simulink model "robot_model_stateflow"  (R2024b)
settings: Solver=FixedStepDiscrete  StartTime=0.0  StopTime=10.0  FixedStep=0.1  RelTol=1e-3  EnableMultiTasking=on
settings Model: Creator=ahmed  LastModifiedBy=ahmed
settings SolverCC: AlgebraicLoopSolver=TrustRegion  AutoInsertRateTranBlk=on
settings DataIOCC: LimitDataPoints=on
settings OptimizationCC: LifeSpan=inf
settings DebuggingCC: UnconnectedInputMsg=warning  UnconnectedOutputMsg=warning  UnconnectedLineMsg=warning  AllowSymbolicDim=off  SFUnexpectedBacktrackingDiag=warning  SFNoUnconditionalDefaultTransitionDiag=warning  SFExecutionAtInitializationDiag=none  ArithmeticOperatorsInVariantConditions=warning
settings ModelReferenceCC: EnableRefExpFcnMdlSchedulingChecks=on
settings SFSimCC: SimUseLocalCustomCode=off  CustomCodeUndefinedFunction=UseInterfaceOnly
settings RTWCC: RTWUseLocalCustomCode=off  GPUComputeCapability=3.5  DLArmComputeVersion=19.05
settings CodeAppCC: StateflowObjectComments=on
settings GRTTargetCC: TargetLangStandard=C89/C90 (ANSI)
settings ConfigComp: CovMetricSettings=dw  CovSaveCumulativeToWorkspaceVar=on  CovSaveSingleToWorkspaceVar=on  CovExternalEMLEnable=off

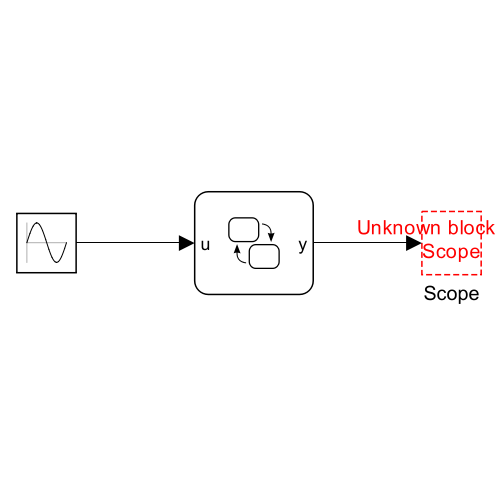
[thumbnail: Simulink's stored preview of the top-level diagram]
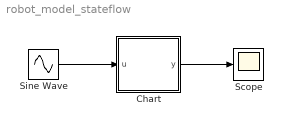
== system robot_model_stateflow ==
  Chart : Stateflow chart  TreatAsAtomicUnit=on
  Scope : Scope
  Sine Wave : Sin  SampleTime=0
  wires:
  Sine Wave/1 -> Chart/1(u)
  Chart/1(y) -> Scope/1

== stateflow chart robot_model_stateflow/Chart ==
  state State4  % Finish
  state State5 %Parking
  state State1 %Ready
  state State2 %Wall tracking
  state state3 %Traffic sign avoidance
  State4  % Finish -> State5 %Parking : [Detected_parking_space == true]
  State2 %Wall tracking -> State4  % Finish [order 2] : [Corner_counter/4 == 3]
  (default) -> State1 %Ready
  State1 %Ready -> State2 %Wall tracking : [button_pressed == 1]
  State2 %Wall tracking -> state3 %Traffic sign avoidance [order 1] : [Saw_traffic_sign == true]
  state3 %Traffic sign avoidance -> State2 %Wall tracking : [Saw_traffic_sign == false]
  data: u input; y output
